simulink model "maxRamp_FromWorkspace"  (R2017b)
settings: Solver=VariableStepAuto  StartTime=0.0  StopTime=10  RelTol=1e-3  EnableMultiTasking=on
undefined symbols (not defined in the file): D_prime, H, P_loss, R, T_d
libraries: simulink x1
settings Model: Creator=lb2916  LastModifiedBy=Luis
settings OptimizationCC: LifeSpan=inf
settings DebuggingCC: SFUnexpectedBacktrackingDiag=warning  SFNoUnconditionalDefaultTransitionDiag=warning  SFExecutionAtInitializationDiag=none
settings CodeAppCC: StateflowObjectComments=on
settings GRTTargetCC: TargetLangStandard=C89/C90 (ANSI)  GeneratePreprocessorConditionals=Disable all
settings ConfigComp: CovMetricSettings=dw  CovHtmlReporting=on  CovSaveCumulativeToWorkspaceVar=on  CovSaveSingleToWorkspaceVar=on  CovExternalEMLEnable=off

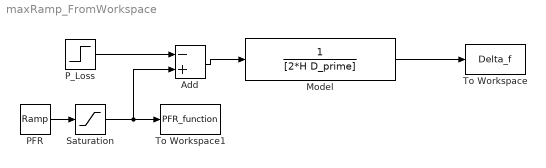
== system maxRamp_FromWorkspace ==
  Add : Sum  Inputs=-+
  Model : TransferFcn  Denominator=[2*H D_prime]
  PFR : simulink/Sources/Ramp  slope=R/T_d  start=0  X0=0
  P_Loss : Step  Time=1000  Before=P_loss  After=P_loss  SampleTime=0
  Saturation : Saturate  UpperLimit=R  LowerLimit=0
  To Workspace : ToWorkspace  VariableName=Delta_f  SaveFormat=Timeseries  SampleTime=-1
  To Workspace1 : ToWorkspace  VariableName=PFR_function  SaveFormat=Timeseries  SampleTime=-1
  wires:
  P_Loss/1 -> Add/1
  Model/1 -> To Workspace/1
  Add/1 -> Model/1
  PFR/1 -> Saturation/1
  Saturation/1 -> To Workspace1/1, Add/2
